simulink model "Linear_model_v2"  (R2021b)
settings: Solver=VariableStepAuto  StartTime=0.0  StopTime=10  MaxStep=1e-6  RelTol=1e-4
values from neighbouring files (symbols this model uses):
  Ipk = Ib*sqrt(2)    [SG_param.m]
  SS_SG = connect(rl_ss,isnb_ss,snb_ss,sg,vsg_pu,vsg,exf,exc_ss,gov_ss,turb_ss,isg_pu,wsg_pu,ang,dang,vgx_g,igx_g,input_vars,output_vars)    [SS_model.m]    (also in SS_model_pu.m = connect(tr_ss,isnb_ss,snb_ss,sg,vsg_pu,vsg,exf,exc_ss,gov_ss)
  Ssg = 50e6    (= 50000000)    [SG_param.m]    (also in sg_slack_POD.m = T_XX.Sb*1e6)
  wn = 2*pi*fn    (= 314.159265359)    [SG_param.m]
settings Model: Creator=Collados  LastModifiedBy=Collados
settings SolverCC: AlgebraicLoopSolver=TrustRegion
settings DebuggingCC: SFMachineParentedDataDiag=warning

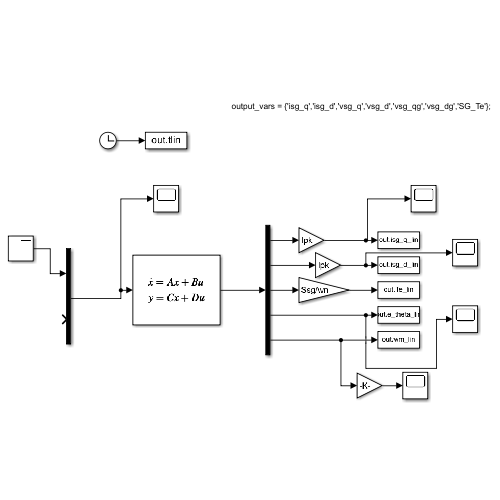
[thumbnail: Simulink's stored preview of the top-level diagram]
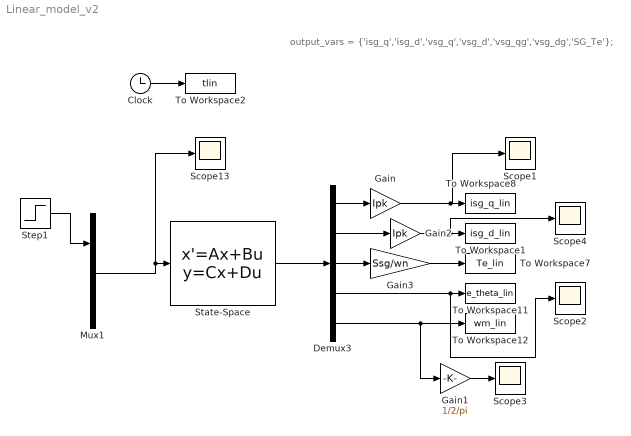
== system Linear_model_v2 ==
  note: output_vars = {'isg_q','isg_d','vsg_q','vsg_d','vsg_qg','vsg_dg','SG_Te'};
  Clock : Clock
  Demux3 : Demux  Outputs=5
  Gain : Gain  Gain=Ipk
  Gain1 : Gain  Gain=1/2/pi
  Gain2 : Gain  Gain=Ipk
  Gain3 : Gain  Gain=Ssg/wn
  Mux1 : Mux  Inputs=length(SS_SG.InputName)
  Scope{1..4,13} (5 alike) : Scope
  State-Space : StateSpace  A=SS_SG.A  B=SS_SG.B  C=SS_SG.C  D=SS_SG.D  InitialCondition=zeros(length(SS_SG.A),1)
  Step1 : Step  After=0.005  SampleTime=0
  To Workspace1 : ToWorkspace  VariableName=isg_d_lin  SampleTime=-1
      settings: Decimation=20  Save2DSignal=2-D array (concatenate along first dimension)
  To Workspace11 : ToWorkspace  VariableName=e_theta_lin  SampleTime=-1
      settings: Decimation=20  Save2DSignal=2-D array (concatenate along first dimension)
  To Workspace12 : ToWorkspace  VariableName=wm_lin  SampleTime=-1
      settings: Decimation=20  Save2DSignal=2-D array (concatenate along first dimension)
  To Workspace2 : ToWorkspace  VariableName=tlin  SampleTime=-1
      settings: Decimation=20  Save2DSignal=2-D array (concatenate along first dimension)
  To Workspace7 : ToWorkspace  VariableName=Te_lin  SampleTime=-1
      settings: Decimation=20  Save2DSignal=2-D array (concatenate along first dimension)
  To Workspace8 : ToWorkspace  VariableName=isg_q_lin  SampleTime=-1
      settings: Decimation=20  Save2DSignal=2-D array (concatenate along first dimension)
  wires:
  Mux1/1 -> Scope13/1, State-Space/1
  State-Space/1 -> Demux3/1
  Step1/1 -> Mux1/1
  Clock/1 -> To Workspace2/1
  Demux3/1 -> Gain/1
  Demux3/2 -> Gain2/1
  Demux3/3 -> Gain3/1
  Demux3/4 -> Scope2/1, To Workspace11/1
  Demux3/5 -> Gain1/1, To Workspace12/1
  Gain/1 -> Scope1/1, To Workspace8/1
  Gain1/1 -> Scope3/1
  Gain2/1 -> Scope4/1, To Workspace1/1
  Gain3/1 -> To Workspace7/1
